simulink model "SISO_Example_Sim"  (R2017b)
settings: Solver=ode3  StartTime=0.0  StopTime=tfin  FixedStep=dT  RelTol=1e-3
values from neighbouring files (symbols this model uses):
  A = [-a_p, b_p, 0, 0 ... (first row only)    [SISO_Example.m]    (also in SimVFA.m = A')
  a20 = 1    [SISO_Example.m]
  a21 = 2    [SISO_Example.m]
  a22 = 1    [SISO_Example.m]
  A_cmd = [0,   1 ... (first row only)    [SISO_Example.m]
  A_h = [0,   1 ... (first row only)    [SISO_Example.m]
  A_m = A - b_3 * k'    [SISO_Example.m]
  A_star = A + b_1*psi_star_1' + b_3*psi_star_3'    [SISO_Example.m]
  adapt = 1    [SISO_Example.m]
  B_cmd = [0; om_cmd^2]    [SISO_Example.m]
  b_h = [0; a20/a22]    [SISO_Example.m]
  b_p = 1.5    [SISO_Example.m]
  b_r = [0; 0; 0; -1]    [SISO_Example.m]
  ba_2 = a22 * A * b_3 + a21 * b_3    [SISO_Example.m]
  ba_3 = a22 * b_3    [SISO_Example.m]
  C_cmd = eye(2)    [SISO_Example.m]
  c_h1 = [0; 1]    [SISO_Example.m]
  c_h2 = [-a20/a22; -a21/a22]    [SISO_Example.m]
  cmd_mag = 1    [SISO_Example.m]
  g = 32.2    [VFA_v1.m]
  k = lqr(A, b_3, Q, r)'    [SISO_Example.m]
  l = eps * ba_1 * b_p * om_n^2    [SISO_Example.m]
  lam_star = lam_star_p * lam_star_a    (= 1)    [SISO_Example.m]
  mu = 2    [SISO_Example.m]
  om_n = 2.6    [SISO_Example.m]
  sine_freq = 1    [SISO_Example.m]
  step_time = 1    [SISO_Example.m]
  steps = length(so.tout)    [SISO_Example.m]    (also in SimVFA.m = length(SOO.t_sim))
settings Model: Creator=ben  LastModifiedBy=ben
settings DataIOCC: SaveOutput=off  SignalLogging=off  DSMLogging=off  ReturnWorkspaceOutputs=on  ReturnWorkspaceOutputsName=simout

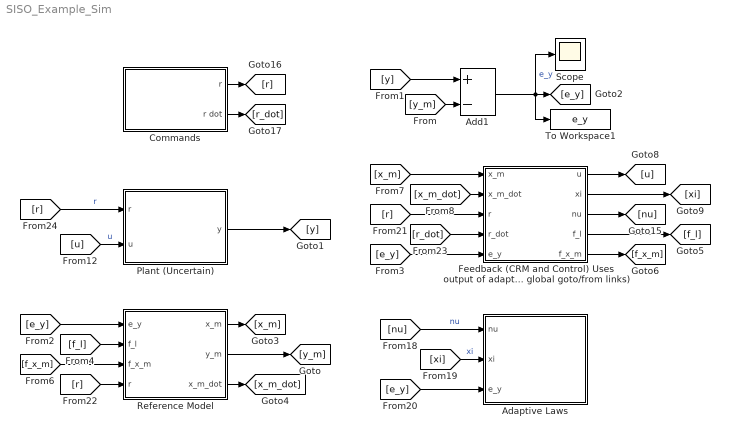
== system SISO_Example_Sim ==
  Adaptive Laws : Subsystem
  Add1 : Sum  Inputs=+-
  Commands : Subsystem
  Feedback (CRM and Control) Uses output of adaptive laws (here via global goto/from links) : Subsystem
  Plant (Uncertain) : Subsystem
  Reference Model : Subsystem
  Scope : Scope
  To Workspace1 : ToWorkspace  VariableName=e_y  SampleTime=-1
  wires:
  [y] -> Add1/1
  [y_m] -> Add1/2
  Add1/1 -> Scope/1, To Workspace1/1, [e_y]  "e_y"
  [e_y] -> Reference Model/1(e_y)
  Reference Model/1(x_m) -> [x_m]
  Reference Model/2(y_m) -> [y_m]
  Reference Model/3(x_m_dot) -> [x_m_dot]
  [f_l] -> Reference Model/2(f_l)
  [f_x_m] -> Reference Model/3(f_x_m)
  [nu] -> Adaptive Laws/1(nu)  "nu"
  [xi] -> Adaptive Laws/2(xi)  "xi"
  [e_y] -> Adaptive Laws/3(e_y)
  Commands/1(r) -> [r]
  Commands/2(r dot) -> [r_dot]
  [r] -> Reference Model/4(r)
  [r] -> Plant (Uncertain)/1(r)  "r"
  [u] -> Plant (Uncertain)/2(u)  "u"
  Plant (Uncertain)/1(y) -> [y]
  [x_m] -> Feedback (CRM and Control) Uses output of adaptive laws (here via global goto/from links)/1(x_m)
  [x_m_dot] -> Feedback (CRM and Control) Uses output of adaptive laws (here via global goto/from links)/2(x_m_dot)
  [r] -> Feedback (CRM and Control) Uses output of adaptive laws (here via global goto/from links)/3(r)
  [r_dot] -> Feedback (CRM and Control) Uses output of adaptive laws (here via global goto/from links)/4(r_dot)
  [e_y] -> Feedback (CRM and Control) Uses output of adaptive laws (here via global goto/from links)/5(e_y)
  Feedback (CRM and Control) Uses output of adaptive laws (here via global goto/from links)/1(u) -> [u]
  Feedback (CRM and Control) Uses output of adaptive laws (here via global goto/from links)/2(xi) -> [xi]
  Feedback (CRM and Control) Uses output of adaptive laws (here via global goto/from links)/3(nu) -> [nu]
  Feedback (CRM and Control) Uses output of adaptive laws (here via global goto/from links)/4(f_l) -> [f_l]
  Feedback (CRM and Control) Uses output of adaptive laws (here via global goto/from links)/5(f_x_m) -> [f_x_m]

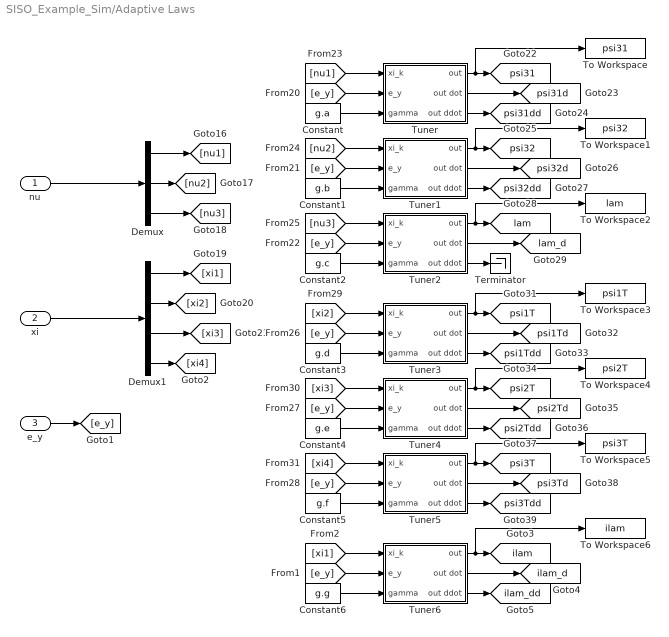
== system SISO_Example_Sim/Adaptive Laws ==
  nu : Inport
  xi : Inport  Port=2
  e_y : Inport  Port=3
  Constant : Constant  Value=g.a
  Constant1 : Constant  Value=g.b
  Constant2 : Constant  Value=g.c
  Constant3 : Constant  Value=g.d
  Constant4 : Constant  Value=g.e
  Constant5 : Constant  Value=g.f
  Constant6 : Constant  Value=g.g
  Demux : Demux  Outputs=[1 1 1]
  Demux1 : Demux  Outputs=[1 4 4 4]
  Terminator : Terminator
  To Workspace : ToWorkspace  VariableName=psi31  SampleTime=-1
  To Workspace1 : ToWorkspace  VariableName=psi32  SampleTime=-1
  To Workspace2 : ToWorkspace  VariableName=lam  SampleTime=-1
  To Workspace3 : ToWorkspace  VariableName=psi1T  SampleTime=-1
  To Workspace4 : ToWorkspace  VariableName=psi2T  SampleTime=-1
  To Workspace5 : ToWorkspace  VariableName=psi3T  SampleTime=-1
  To Workspace6 : ToWorkspace  VariableName=ilam  SampleTime=-1
  Tuner : Subsystem
  Tuner1 : Subsystem
  Tuner2 : Subsystem
  Tuner3 : Subsystem
  Tuner4 : Subsystem
  Tuner5 : Subsystem
  Tuner6 : Subsystem
  tag scope: ilam=global, ilam_d=global, ilam_dd=global, lam=global, lam_d=global, psi1T=global, psi1Td=global, psi1Tdd=global, psi2T=global, psi2Td=global, psi2Tdd=global, psi31=global, psi31d=global, psi31dd=global, psi32=global, psi32d=global, psi32dd=global, psi3T=global, psi3Td=global, psi3Tdd=global
  wires:
  Tuner3/3(out ddot) -> [psi1Tdd]
  nu/1 -> Demux/1
  Tuner5/2(out dot) -> [psi3Td]
  Demux/1 -> [nu1]
  Tuner4/1(out) -> To Workspace4/1, [psi2T]
  [nu1] -> Tuner/1(xi_k)
  [nu2] -> Tuner1/1(xi_k)
  [e_y] -> Tuner1/2(e_y)
  [e_y] -> Tuner/2(e_y)
  Tuner2/1(out) -> To Workspace2/1, [lam]
  Tuner/3(out ddot) -> [psi31dd]
  Tuner1/3(out ddot) -> [psi32dd]
  Tuner3/1(out) -> To Workspace3/1, [psi1T]
  Demux/3 -> [nu3]
  [xi4] -> Tuner5/1(xi_k)
  [e_y] -> Tuner3/2(e_y)
  Tuner/2(out dot) -> [psi31d]
  Tuner1/2(out dot) -> [psi32d]
  [xi2] -> Tuner3/1(xi_k)
  [e_y] -> Tuner5/2(e_y)
  [e_y] -> Tuner4/2(e_y)
  [xi3] -> Tuner4/1(xi_k)
  xi/1 -> Demux1/1
  [e_y] -> Tuner2/2(e_y)
  Tuner2/3(out ddot) -> Terminator/1
  Demux1/3 -> [xi3]
  Tuner5/3(out ddot) -> [psi3Tdd]
  [nu3] -> Tuner2/1(xi_k)
  Tuner/1(out) -> To Workspace/1, [psi31]
  Tuner2/2(out dot) -> [lam_d]
  Tuner4/2(out dot) -> [psi2Td]
  Tuner1/1(out) -> To Workspace1/1, [psi32]
  Tuner4/3(out ddot) -> [psi2Tdd]
  Demux1/1 -> [xi1]
  Demux1/2 -> [xi2]
  Demux/2 -> [nu2]
  Tuner3/2(out dot) -> [psi1Td]
  e_y/1 -> [e_y]
  Tuner5/1(out) -> To Workspace5/1, [psi3T]
  Demux1/4 -> [xi4]
  [xi1] -> Tuner6/1(xi_k)
  [e_y] -> Tuner6/2(e_y)
  Tuner6/1(out) -> To Workspace6/1, [ilam]
  Tuner6/3(out ddot) -> [ilam_dd]
  Tuner6/2(out dot) -> [ilam_d]
  Constant/1 -> Tuner/3(gamma)
  Constant1/1 -> Tuner1/3(gamma)
  Constant2/1 -> Tuner2/3(gamma)
  Constant3/1 -> Tuner3/3(gamma)
  Constant4/1 -> Tuner4/3(gamma)
  Constant5/1 -> Tuner5/3(gamma)
  Constant6/1 -> Tuner6/3(gamma)

== system SISO_Example_Sim/Commands ==
  Command Filter : StateSpace  A=A_cmd  B=B_cmd  C=C_cmd  D=[0; 0]  InitialCondition=0
  Constant : Constant  Value=steps
  Constant1 : Constant  Value=cmd_mag/2
  Demux : Demux  Outputs=[1 1]
  Pulse Generator : DiscretePulseGenerator  PulseType=Time based  Amplitude=cmd_mag  Period=2*step_time  PulseWidth=50
  Sine Wave : Sin  Amplitude=cmd_mag  Frequency=sine_freq  SampleTime=0
  Sum : Sum  Inputs=-+|
  Switch : Switch  Criteria=u2 ~= 0
  To Workspace1 : ToWorkspace  VariableName=r_dot  SampleTime=-1
  To Workspace3 : ToWorkspace  VariableName=r  SampleTime=-1
  r : Outport
  r dot : Outport  Port=2
  wires:
  Demux/2 -> To Workspace1/1, r dot/1  "r dot"
  Command Filter/1 -> Demux/1
  Demux/1 -> To Workspace3/1, r/1  "r (alternatively z_cmd)"
  Constant/1 -> Switch/2
  Switch/1 -> Command Filter/1
  Sum/1 -> Switch/1
  Sine Wave/1 -> Switch/3
  Pulse Generator/1 -> Sum/2
  Constant1/1 -> Sum/1

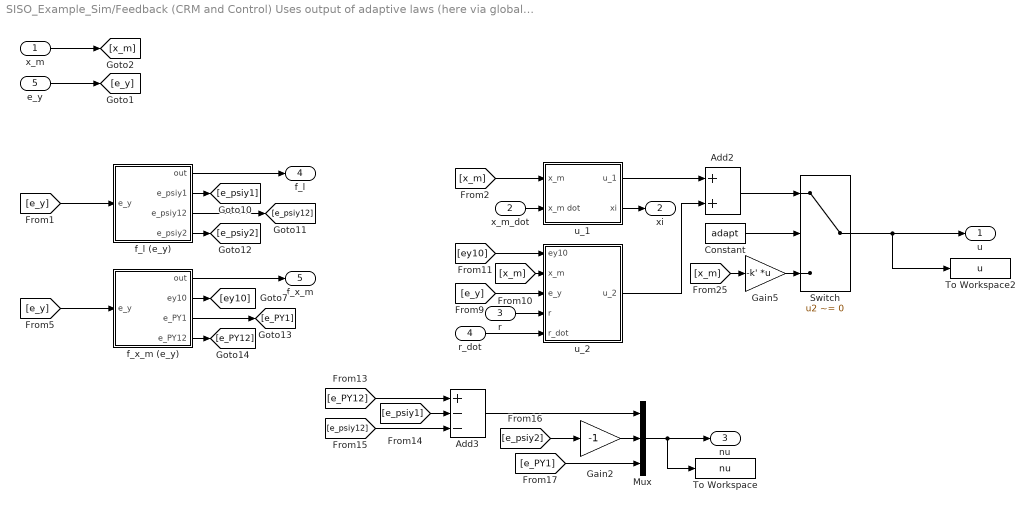
== system SISO_Example_Sim/Feedback (CRM and Control) Uses output of adaptive laws (here via global goto//from links) ==
  x_m : Inport
  x_m_dot : Inport  Port=2
  r : Inport  Port=3
  r_dot : Inport  Port=4
  e_y : Inport  Port=5
  Add2 : Sum
  Add3 : Sum  Inputs=+--
  Constant : Constant  Value=adapt
  Gain2 : Gain  Gain=-1
  Gain5 : Gain  Gain=-k'  Multiplication=Matrix(K*u)
  Mux : Mux  Inputs=[1 1 1]
  Switch : Switch  Criteria=u2 ~= 0
  To Workspace : ToWorkspace  VariableName=nu  SampleTime=-1
  To Workspace2 : ToWorkspace  VariableName=u  SampleTime=-1
  f_l (e_y) : Subsystem
  f_x_m (e_y) : Subsystem
  u_1 : Subsystem
  u_2 : Subsystem
  u : Outport
  xi : Outport  Port=2
  nu : Outport  Port=3
  f_l : Outport  Port=4
  f_x_m : Outport  Port=5
  wires:
  [e_PY1] -> Mux/3
  Gain2/1 -> Mux/2
  [e_psiy2] -> Gain2/1
  [e_psiy12] -> Add3/3
  [e_psiy1] -> Add3/2
  [e_PY12] -> Add3/1
  Add3/1 -> Mux/1
  f_x_m (e_y)/4(e_PY12) -> [e_PY12]
  f_x_m (e_y)/3(e_PY1) -> [e_PY1]
  f_l (e_y)/4(e_psiy2) -> [e_psiy2]
  f_l (e_y)/3(e_psiy12) -> [e_psiy12]
  f_l (e_y)/2(e_psiy1) -> [e_psiy1]
  u_1/2(xi) -> xi/1
  Switch/1 -> u/1, To Workspace2/1
  u_2/1(u_2) -> Add2/2
  u_1/1(u_1) -> Add2/1
  [ey10] -> u_2/1(ey10)
  [e_y] -> u_2/3(e_y)
  f_x_m (e_y)/2(ey10) -> [ey10]
  x_m_dot/1 -> u_1/2(x_m dot)
  f_x_m (e_y)/1(out) -> f_x_m/1
  [e_y] -> f_x_m (e_y)/1(e_y)
  [x_m] -> u_2/2(x_m)
  f_l (e_y)/1(out) -> f_l/1
  Mux/1 -> nu/1, To Workspace/1
  r/1 -> u_2/4(r)
  r_dot/1 -> u_2/5(r_dot)
  Constant/1 -> Switch/2
  Add2/1 -> Switch/1
  Gain5/1 -> Switch/3
  [x_m] -> Gain5/1
  e_y/1 -> [e_y]
  [e_y] -> f_l (e_y)/1(e_y)
  x_m/1 -> [x_m]
  [x_m] -> u_1/1(x_m)

== system SISO_Example_Sim/Plant (Uncertain) ==
  r : Inport
  u : Inport  Port=2
  Add : Sum  Inputs=+++
  Gain1 : Gain  Gain=lam_star
  Gain3 : Gain  Gain=b_r  Multiplication=Matrix(K*u)
  Gain4 : Gain  Gain=A_star  Multiplication=Matrix(K*u)
  Gain5 : Gain  Gain=c'  Multiplication=Matrix(K*u)
  Integrator : Integrator
  Signal Specification2 : SignalSpecification  Dimensions=[4 1]
  To Workspace3 : ToWorkspace  VariableName=y  SampleTime=-1
  y : Outport
  wires:
  u/1 -> Gain1/1
  Gain5/1 -> y/1, To Workspace3/1
  Add/1 -> Signal Specification2/1  "x_dot"
  Gain4/1 -> Add/1  "(A*) * x"
  Integrator/1 -> Gain4/1, Gain5/1  "x"
  Gain3/1 -> Add/2  "b_r * r"
  r/1 -> Gain3/1
  Signal Specification2/1 -> Integrator/1  "x_dot"
  Gain1/1 -> Add/3

== system SISO_Example_Sim/Reference Model ==
  e_y : Inport
  f_l : Inport  Port=2
  f_x_m : Inport  Port=3
  r : Inport  Port=4
  Add : Sum  Inputs=+++++
  Gain : Gain  Gain=c'  Multiplication=Matrix(K*u)
  Gain1 : Gain  Gain=l  Multiplication=Matrix(K*u)
  Gain2 : Gain  Gain=A_m  Multiplication=Matrix(K*u)
  Gain3 : Gain  Gain=b_r  Multiplication=Matrix(K*u)
  Integrator : Integrator
  Signal Specification2 : SignalSpecification  Dimensions=[4 1]
  To Workspace : ToWorkspace  VariableName=x_m  SampleTime=-1
  To Workspace1 : ToWorkspace  VariableName=y_m  SampleTime=-1
  x_m : Outport
  y_m : Outport  Port=2
  x_m_dot : Outport  Port=3
  wires:
  Gain2/1 -> Add/1  "A_m * x_m"
  f_x_m/1 -> Add/4
  e_y/1 -> Gain1/1
  Gain/1 -> To Workspace1/1, y_m/1  "y_m"
  Gain1/1 -> Add/2  "l * e_y"
  Integrator/1 -> To Workspace/1, x_m/1, Gain2/1, Gain/1  "x_m"
  Signal Specification2/1 -> x_m_dot/1, Integrator/1  "x_m_dot"
  f_l/1 -> Add/3
  Add/1 -> Signal Specification2/1  "x_m_dot"
  Gain3/1 -> Add/5
  r/1 -> Gain3/1

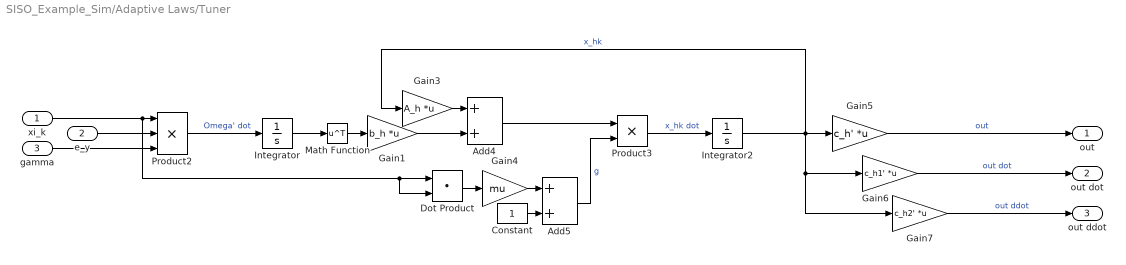
== system SISO_Example_Sim/Adaptive Laws/Tuner ==
  xi_k : Inport
  e_y : Inport  Port=2
  gamma : Inport  Port=3
  Add4 : Sum
  Add5 : Sum
  Constant : Constant
  Dot Product : DotProduct  InputSameDT=on  OutDataTypeStr=Inherit: Inherit via internal rule
  Gain1 : Gain  Gain=b_h  Multiplication=Matrix(K*u)
  Gain3 : Gain  Gain=A_h  Multiplication=Matrix(K*u)
  Gain4 : Gain  Gain=mu
  Gain5 : Gain  Gain=c_h'  Multiplication=Matrix(K*u)
  Gain6 : Gain  Gain=c_h1'  Multiplication=Matrix(K*u)
  Gain7 : Gain  Gain=c_h2'  Multiplication=Matrix(K*u)
  Integrator : Integrator
  Integrator2 : Integrator
  Math Function : Math  Operator=transpose  SaturateOnIntegerOverflow=on
  Product2 : Product  Inputs=3
  Product3 : Product
  out : Outport
  out dot : Outport  Port=2
  out ddot : Outport  Port=3
  wires:
  Constant/1 -> Add5/2
  Math Function/1 -> Gain1/1
  Add4/1 -> Product3/1
  e_y/1 -> Product2/2
  Gain5/1 -> out/1  "out"
  Gain1/1 -> Add4/2
  Product3/1 -> Integrator2/1  "x_hk dot"
  Integrator/1 -> Math Function/1
  Integrator2/1 -> Gain7/1, Gain6/1, Gain5/1, Gain3/1  "x_hk"
  Gain7/1 -> out ddot/1  "out ddot"
  Product2/1 -> Integrator/1  "Omega' dot"
  Add5/1 -> Product3/2  "g"
  xi_k/1 -> Dot Product/2, Dot Product/1, Product2/1
  Gain4/1 -> Add5/1
  Dot Product/1 -> Gain4/1
  Gain3/1 -> Add4/1
  Gain6/1 -> out dot/1  "out dot"
  gamma/1 -> Product2/3

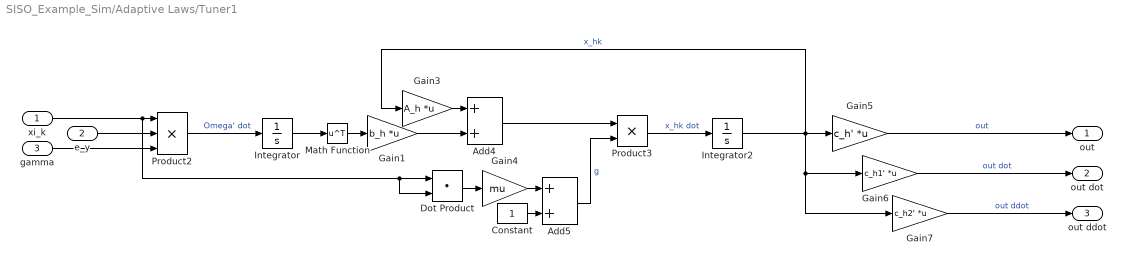
== system SISO_Example_Sim/Adaptive Laws/Tuner1 ==
  xi_k : Inport
  e_y : Inport  Port=2
  gamma : Inport  Port=3
  Add4 : Sum
  Add5 : Sum
  Constant : Constant
  Dot Product : DotProduct  InputSameDT=on  OutDataTypeStr=Inherit: Inherit via internal rule
  Gain1 : Gain  Gain=b_h  Multiplication=Matrix(K*u)
  Gain3 : Gain  Gain=A_h  Multiplication=Matrix(K*u)
  Gain4 : Gain  Gain=mu
  Gain5 : Gain  Gain=c_h'  Multiplication=Matrix(K*u)
  Gain6 : Gain  Gain=c_h1'  Multiplication=Matrix(K*u)
  Gain7 : Gain  Gain=c_h2'  Multiplication=Matrix(K*u)
  Integrator : Integrator
  Integrator2 : Integrator
  Math Function : Math  Operator=transpose  SaturateOnIntegerOverflow=on
  Product2 : Product  Inputs=3
  Product3 : Product
  out : Outport
  out dot : Outport  Port=2
  out ddot : Outport  Port=3
  wires:
  gamma/1 -> Product2/3
  Gain6/1 -> out dot/1  "out dot"
  Gain3/1 -> Add4/1
  Dot Product/1 -> Gain4/1
  Gain4/1 -> Add5/1
  xi_k/1 -> Product2/1, Dot Product/1, Dot Product/2
  Add5/1 -> Product3/2  "g"
  Product2/1 -> Integrator/1  "Omega' dot"
  Gain7/1 -> out ddot/1  "out ddot"
  Integrator2/1 -> Gain3/1, Gain5/1, Gain6/1, Gain7/1  "x_hk"
  Integrator/1 -> Math Function/1
  Product3/1 -> Integrator2/1  "x_hk dot"
  Gain1/1 -> Add4/2
  Gain5/1 -> out/1  "out"
  e_y/1 -> Product2/2
  Add4/1 -> Product3/1
  Math Function/1 -> Gain1/1
  Constant/1 -> Add5/2

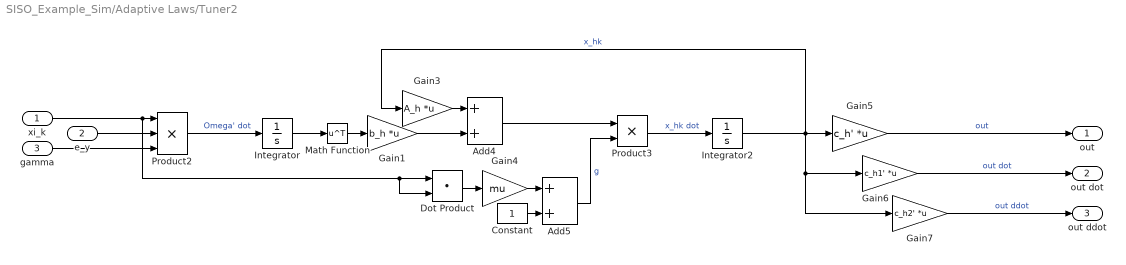
== system SISO_Example_Sim/Adaptive Laws/Tuner2 ==
  xi_k : Inport
  e_y : Inport  Port=2
  gamma : Inport  Port=3
  Add4 : Sum
  Add5 : Sum
  Constant : Constant
  Dot Product : DotProduct  InputSameDT=on  OutDataTypeStr=Inherit: Inherit via internal rule
  Gain1 : Gain  Gain=b_h  Multiplication=Matrix(K*u)
  Gain3 : Gain  Gain=A_h  Multiplication=Matrix(K*u)
  Gain4 : Gain  Gain=mu
  Gain5 : Gain  Gain=c_h'  Multiplication=Matrix(K*u)
  Gain6 : Gain  Gain=c_h1'  Multiplication=Matrix(K*u)
  Gain7 : Gain  Gain=c_h2'  Multiplication=Matrix(K*u)
  Integrator : Integrator
  Integrator2 : Integrator  InitialCondition=[1; 0]
  Math Function : Math  Operator=transpose  SaturateOnIntegerOverflow=on
  Product2 : Product  Inputs=3
  Product3 : Product
  out : Outport
  out dot : Outport  Port=2
  out ddot : Outport  Port=3
  wires:
  Constant/1 -> Add5/2
  Math Function/1 -> Gain1/1
  Add4/1 -> Product3/1
  e_y/1 -> Product2/2
  Gain5/1 -> out/1  "out"
  Gain1/1 -> Add4/2
  Product3/1 -> Integrator2/1  "x_hk dot"
  Integrator/1 -> Math Function/1
  Integrator2/1 -> Gain7/1, Gain6/1, Gain5/1, Gain3/1  "x_hk"
  Gain7/1 -> out ddot/1  "out ddot"
  Product2/1 -> Integrator/1  "Omega' dot"
  Add5/1 -> Product3/2  "g"
  xi_k/1 -> Dot Product/2, Dot Product/1, Product2/1
  Gain4/1 -> Add5/1
  Dot Product/1 -> Gain4/1
  Gain3/1 -> Add4/1
  Gain6/1 -> out dot/1  "out dot"
  gamma/1 -> Product2/3

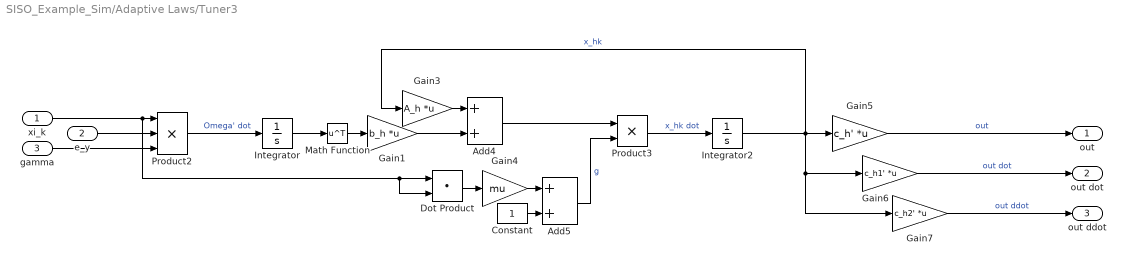
== system SISO_Example_Sim/Adaptive Laws/Tuner3 ==
  xi_k : Inport
  e_y : Inport  Port=2
  gamma : Inport  Port=3
  Add4 : Sum
  Add5 : Sum
  Constant : Constant
  Dot Product : DotProduct  InputSameDT=on  OutDataTypeStr=Inherit: Inherit via internal rule
  Gain1 : Gain  Gain=b_h  Multiplication=Matrix(K*u)
  Gain3 : Gain  Gain=A_h  Multiplication=Matrix(K*u)
  Gain4 : Gain  Gain=mu
  Gain5 : Gain  Gain=c_h'  Multiplication=Matrix(K*u)
  Gain6 : Gain  Gain=c_h1'  Multiplication=Matrix(K*u)
  Gain7 : Gain  Gain=c_h2'  Multiplication=Matrix(K*u)
  Integrator : Integrator
  Integrator2 : Integrator
  Math Function : Math  Operator=transpose  SaturateOnIntegerOverflow=on
  Product2 : Product  Inputs=3
  Product3 : Product
  out : Outport
  out dot : Outport  Port=2
  out ddot : Outport  Port=3
  wires:
  gamma/1 -> Product2/3
  Gain6/1 -> out dot/1  "out dot"
  Gain3/1 -> Add4/1
  Dot Product/1 -> Gain4/1
  Gain4/1 -> Add5/1
  xi_k/1 -> Product2/1, Dot Product/1, Dot Product/2
  Add5/1 -> Product3/2  "g"
  Product2/1 -> Integrator/1  "Omega' dot"
  Gain7/1 -> out ddot/1  "out ddot"
  Integrator2/1 -> Gain3/1, Gain5/1, Gain6/1, Gain7/1  "x_hk"
  Integrator/1 -> Math Function/1
  Product3/1 -> Integrator2/1  "x_hk dot"
  Gain1/1 -> Add4/2
  Gain5/1 -> out/1  "out"
  e_y/1 -> Product2/2
  Add4/1 -> Product3/1
  Math Function/1 -> Gain1/1
  Constant/1 -> Add5/2

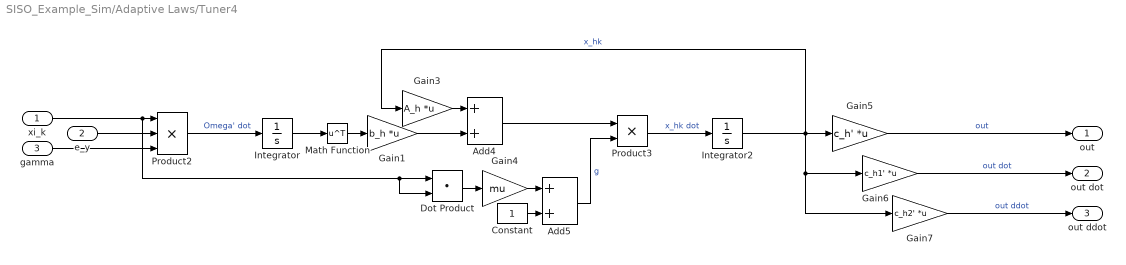
== system SISO_Example_Sim/Adaptive Laws/Tuner4 ==
  xi_k : Inport
  e_y : Inport  Port=2
  gamma : Inport  Port=3
  Add4 : Sum
  Add5 : Sum
  Constant : Constant
  Dot Product : DotProduct  InputSameDT=on  OutDataTypeStr=Inherit: Inherit via internal rule
  Gain1 : Gain  Gain=b_h  Multiplication=Matrix(K*u)
  Gain3 : Gain  Gain=A_h  Multiplication=Matrix(K*u)
  Gain4 : Gain  Gain=mu
  Gain5 : Gain  Gain=c_h'  Multiplication=Matrix(K*u)
  Gain6 : Gain  Gain=c_h1'  Multiplication=Matrix(K*u)
  Gain7 : Gain  Gain=c_h2'  Multiplication=Matrix(K*u)
  Integrator : Integrator
  Integrator2 : Integrator
  Math Function : Math  Operator=transpose  SaturateOnIntegerOverflow=on
  Product2 : Product  Inputs=3
  Product3 : Product
  out : Outport
  out dot : Outport  Port=2
  out ddot : Outport  Port=3
  wires:
  Constant/1 -> Add5/2
  Math Function/1 -> Gain1/1
  Add4/1 -> Product3/1
  e_y/1 -> Product2/2
  Gain5/1 -> out/1  "out"
  Gain1/1 -> Add4/2
  Product3/1 -> Integrator2/1  "x_hk dot"
  Integrator/1 -> Math Function/1
  Integrator2/1 -> Gain7/1, Gain6/1, Gain5/1, Gain3/1  "x_hk"
  Gain7/1 -> out ddot/1  "out ddot"
  Product2/1 -> Integrator/1  "Omega' dot"
  Add5/1 -> Product3/2  "g"
  xi_k/1 -> Dot Product/2, Dot Product/1, Product2/1
  Gain4/1 -> Add5/1
  Dot Product/1 -> Gain4/1
  Gain3/1 -> Add4/1
  Gain6/1 -> out dot/1  "out dot"
  gamma/1 -> Product2/3

== system SISO_Example_Sim/Adaptive Laws/Tuner5 ==
  xi_k : Inport
  e_y : Inport  Port=2
  gamma : Inport  Port=3
  Add4 : Sum
  Add5 : Sum
  Constant : Constant
  Dot Product : DotProduct  InputSameDT=on  OutDataTypeStr=Inherit: Inherit via internal rule
  Gain1 : Gain  Gain=b_h  Multiplication=Matrix(K*u)
  Gain3 : Gain  Gain=A_h  Multiplication=Matrix(K*u)
  Gain4 : Gain  Gain=mu
  Gain5 : Gain  Gain=c_h'  Multiplication=Matrix(K*u)
  Gain6 : Gain  Gain=c_h1'  Multiplication=Matrix(K*u)
  Gain7 : Gain  Gain=c_h2'  Multiplication=Matrix(K*u)
  Integrator : Integrator
  Integrator2 : Integrator
  Math Function : Math  Operator=transpose  SaturateOnIntegerOverflow=on
  Product2 : Product  Inputs=3
  Product3 : Product
  out : Outport
  out dot : Outport  Port=2
  out ddot : Outport  Port=3
  wires:
  gamma/1 -> Product2/3
  Gain6/1 -> out dot/1  "out dot"
  Gain3/1 -> Add4/1
  Dot Product/1 -> Gain4/1
  Gain4/1 -> Add5/1
  xi_k/1 -> Product2/1, Dot Product/1, Dot Product/2
  Add5/1 -> Product3/2  "g"
  Product2/1 -> Integrator/1  "Omega' dot"
  Gain7/1 -> out ddot/1  "out ddot"
  Integrator2/1 -> Gain3/1, Gain5/1, Gain6/1, Gain7/1  "x_hk"
  Integrator/1 -> Math Function/1
  Product3/1 -> Integrator2/1  "x_hk dot"
  Gain1/1 -> Add4/2
  Gain5/1 -> out/1  "out"
  e_y/1 -> Product2/2
  Add4/1 -> Product3/1
  Math Function/1 -> Gain1/1
  Constant/1 -> Add5/2

== system SISO_Example_Sim/Adaptive Laws/Tuner6 ==
  xi_k : Inport
  e_y : Inport  Port=2
  gamma : Inport  Port=3
  Add4 : Sum
  Add5 : Sum
  Constant : Constant
  Dot Product : DotProduct  InputSameDT=on  OutDataTypeStr=Inherit: Inherit via internal rule
  Gain1 : Gain  Gain=b_h  Multiplication=Matrix(K*u)
  Gain3 : Gain  Gain=A_h  Multiplication=Matrix(K*u)
  Gain4 : Gain  Gain=mu
  Gain5 : Gain  Gain=c_h'  Multiplication=Matrix(K*u)
  Gain6 : Gain  Gain=c_h1'  Multiplication=Matrix(K*u)
  Gain7 : Gain  Gain=c_h2'  Multiplication=Matrix(K*u)
  Integrator : Integrator
  Integrator2 : Integrator  InitialCondition=[1; 0]
  Math Function : Math  Operator=transpose  SaturateOnIntegerOverflow=on
  Product2 : Product  Inputs=3
  Product3 : Product
  out : Outport
  out dot : Outport  Port=2
  out ddot : Outport  Port=3
  wires:
  Constant/1 -> Add5/2
  Math Function/1 -> Gain1/1
  Add4/1 -> Product3/1
  e_y/1 -> Product2/2
  Gain5/1 -> out/1  "out"
  Gain1/1 -> Add4/2
  Product3/1 -> Integrator2/1  "x_hk dot"
  Integrator/1 -> Math Function/1
  Integrator2/1 -> Gain7/1, Gain6/1, Gain5/1, Gain3/1  "x_hk"
  Gain7/1 -> out ddot/1  "out ddot"
  Product2/1 -> Integrator/1  "Omega' dot"
  Add5/1 -> Product3/2  "g"
  xi_k/1 -> Dot Product/2, Dot Product/1, Product2/1
  Gain4/1 -> Add5/1
  Dot Product/1 -> Gain4/1
  Gain3/1 -> Add4/1
  Gain6/1 -> out dot/1  "out dot"
  gamma/1 -> Product2/3

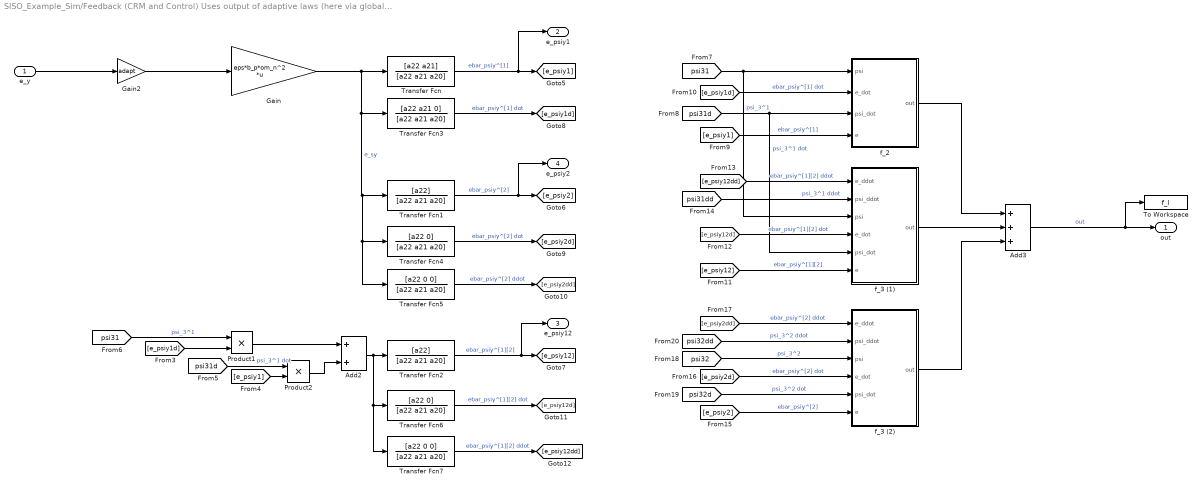
== system SISO_Example_Sim/Feedback (CRM and Control) Uses output of adaptive laws (here via global goto//from links)/f_l (e_y) ==
  e_y : Inport
  Add2 : Sum
  Add3 : Sum  Inputs=+++
  Gain : Gain  Gain=eps*b_p*om_n^2  Multiplication=Matrix(K*u)
  Gain2 : Gain  Gain=adapt
  Product1 : Product
  Product2 : Product
  To Workspace : ToWorkspace  VariableName=f_l  SampleTime=-1
  Transfer Fcn : TransferFcn  Numerator=[a22 a21]  Denominator=[a22 a21 a20]
  Transfer Fcn1 : TransferFcn  Numerator=[a22]  Denominator=[a22 a21 a20]
  Transfer Fcn2 : TransferFcn  Numerator=[a22]  Denominator=[a22 a21 a20]
  Transfer Fcn3 : TransferFcn  Numerator=[a22 a21 0]  Denominator=[a22 a21 a20]
  Transfer Fcn4 : TransferFcn  Numerator=[a22 0]  Denominator=[a22 a21 a20]
  Transfer Fcn5 : TransferFcn  Numerator=[a22 0 0]  Denominator=[a22 a21 a20]
  Transfer Fcn6 : TransferFcn  Numerator=[a22 0]  Denominator=[a22 a21 a20]
  Transfer Fcn7 : TransferFcn  Numerator=[a22 0 0]  Denominator=[a22 a21 a20]
  f_2 : Subsystem
  f_3 (1) : Subsystem
  f_3 (2) : Subsystem
  out : Outport
  e_psiy1 : Outport  Port=2
  e_psiy12 : Outport  Port=3
  e_psiy2 : Outport  Port=4
  wires:
  [e_psiy12dd] -> f_3 (1)/1(e_ddot)  "ebar_psiy^[1][2] ddot"
  Transfer Fcn7/1 -> [e_psiy12dd]  "ebar_psiy^[1][2] ddot"
  f_3 (1)/1(out) -> Add3/2
  [psi31d] -> f_2/3(psi_dot), f_3 (1)/5(psi_dot)  "psi_3^1 dot"
  [psi31] -> f_2/1(psi), f_3 (1)/3(psi)  "psi_3^1"
  f_2/1(out) -> Add3/1
  [psi31] -> Product1/1  "psi_3^1"
  Transfer Fcn1/1 -> e_psiy2/1, [e_psiy2]  "ebar_psiy^[2]"
  [e_psiy2dd] -> f_3 (2)/1(e_ddot)  "ebar_psiy^[2] ddot"
  [psi32dd] -> f_3 (2)/2(psi_ddot)  "psi_3^2 ddot"
  [psi32d] -> f_3 (2)/5(psi_dot)  "psi_3^2 dot"
  [e_psiy12d] -> f_3 (1)/4(e_dot)  "ebar_psiy^[1][2] dot"
  [e_psiy1d] -> f_2/2(e_dot)  "ebar_psiy^[1] dot"
  f_3 (2)/1(out) -> Add3/3
  Transfer Fcn4/1 -> [e_psiy2d]  "ebar_psiy^[2] dot"
  [psi31d] -> Product2/1  "psi_3^1 dot"
  Add3/1 -> To Workspace/1, out/1  "out"
  Transfer Fcn6/1 -> [e_psiy12d]  "ebar_psiy^[1][2] dot"
  Transfer Fcn2/1 -> e_psiy12/1, [e_psiy12]  "ebar_psiy^[1][2]"
  [e_psiy2] -> f_3 (2)/6(e)  "ebar_psiy^[2]"
  Gain/1 -> Transfer Fcn3/1, Transfer Fcn5/1, Transfer Fcn4/1, Transfer Fcn1/1, Transfer Fcn/1  "e_sy"
  Add2/1 -> Transfer Fcn7/1, Transfer Fcn6/1, Transfer Fcn2/1
  [e_psiy1] -> Product2/2
  [psi31dd] -> f_3 (1)/2(psi_ddot)  "psi_3^1 ddot"
  Product1/1 -> Add2/1
  [e_psiy1d] -> Product1/2
  Product2/1 -> Add2/2
  Transfer Fcn3/1 -> [e_psiy1d]  "ebar_psiy^[1] dot"
  [e_psiy12] -> f_3 (1)/6(e)  "ebar_psiy^[1][2]"
  Transfer Fcn/1 -> e_psiy1/1, [e_psiy1]  "ebar_psiy^[1]"
  [psi32] -> f_3 (2)/3(psi)  "psi_3^2"
  [e_psiy2d] -> f_3 (2)/4(e_dot)  "ebar_psiy^[2] dot"
  e_y/1 -> Gain2/1
  [e_psiy1] -> f_2/4(e)  "ebar_psiy^[1]"
  Transfer Fcn5/1 -> [e_psiy2dd]  "ebar_psiy^[2] ddot"
  Gain2/1 -> Gain/1

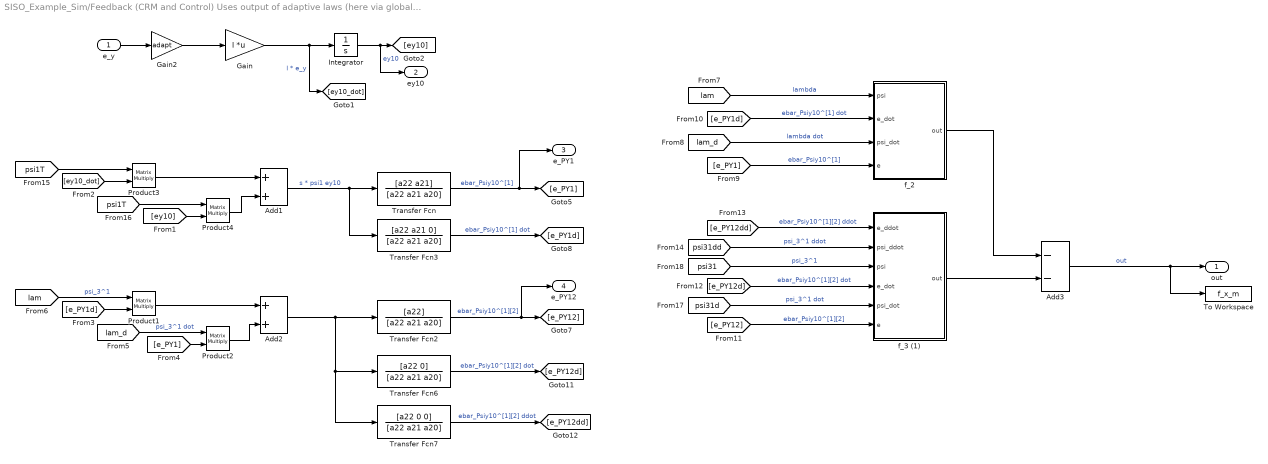
== system SISO_Example_Sim/Feedback (CRM and Control) Uses output of adaptive laws (here via global goto//from links)/f_x_m (e_y) ==
  e_y : Inport
  Add1 : Sum
  Add2 : Sum
  Add3 : Sum  Inputs=--
  Gain : Gain  Gain=l  Multiplication=Matrix(K*u)
  Gain2 : Gain  Gain=adapt
  Integrator : Integrator
  Product{1..4} (4 alike) : Product  Multiplication=Matrix(*)
  To Workspace : ToWorkspace  VariableName=f_x_m  SampleTime=-1
  Transfer Fcn : TransferFcn  Numerator=[a22 a21]  Denominator=[a22 a21 a20]
  Transfer Fcn2 : TransferFcn  Numerator=[a22]  Denominator=[a22 a21 a20]
  Transfer Fcn3 : TransferFcn  Numerator=[a22 a21 0]  Denominator=[a22 a21 a20]
  Transfer Fcn6 : TransferFcn  Numerator=[a22 0]  Denominator=[a22 a21 a20]
  Transfer Fcn7 : TransferFcn  Numerator=[a22 0 0]  Denominator=[a22 a21 a20]
  f_2 : Subsystem
  f_3 (1) : Subsystem
  out : Outport
  ey10 : Outport  Port=2
  e_PY1 : Outport  Port=3
  e_PY12 : Outport  Port=4
  wires:
  [e_PY12dd] -> f_3 (1)/1(e_ddot)  "ebar_Psiy10^[1][2] ddot"
  Transfer Fcn7/1 -> [e_PY12dd]  "ebar_Psiy10^[1][2] ddot"
  f_3 (1)/1(out) -> Add3/2
  [lam_d] -> f_2/3(psi_dot)  "lambda dot"
  [lam] -> f_2/1(psi)  "lambda"
  f_2/1(out) -> Add3/1
  [lam] -> Product1/1  "psi_3^1"
  [e_PY12d] -> f_3 (1)/4(e_dot)  "ebar_Psiy10^[1][2] dot"
  [e_PY1d] -> f_2/2(e_dot)  "ebar_Psiy10^[1] dot"
  [lam_d] -> Product2/1  "psi_3^1 dot"
  Add3/1 -> To Workspace/1, out/1  "out"
  Transfer Fcn6/1 -> [e_PY12d]  "ebar_Psiy10^[1][2] dot"
  Transfer Fcn2/1 -> e_PY12/1, [e_PY12]  "ebar_Psiy10^[1][2]"
  Gain/1 -> [ey10_dot], Integrator/1  "l * e_y"
  Add2/1 -> Transfer Fcn2/1, Transfer Fcn6/1, Transfer Fcn7/1
  [e_PY1] -> Product2/2
  [psi31dd] -> f_3 (1)/2(psi_ddot)  "psi_3^1 ddot"
  Product1/1 -> Add2/1
  [e_PY1d] -> Product1/2
  Product2/1 -> Add2/2
  Transfer Fcn3/1 -> [e_PY1d]  "ebar_Psiy10^[1] dot"
  [e_PY12] -> f_3 (1)/6(e)  "ebar_Psiy10^[1][2]"
  Transfer Fcn/1 -> [e_PY1], e_PY1/1  "ebar_Psiy10^[1]"
  e_y/1 -> Gain2/1
  [e_PY1] -> f_2/4(e)  "ebar_Psiy10^[1]"
  Add1/1 -> Transfer Fcn3/1, Transfer Fcn/1  "s * psi1 ey10"
  Integrator/1 -> ey10/1, [ey10]  "ey10"
  Product4/1 -> Add1/2
  Product3/1 -> Add1/1
  [ey10] -> Product4/2
  [ey10_dot] -> Product3/2
  [psi1T] -> Product3/1
  [psi1T] -> Product4/1
  [psi31d] -> f_3 (1)/5(psi_dot)  "psi_3^1 dot"
  [psi31] -> f_3 (1)/3(psi)  "psi_3^1"
  Gain2/1 -> Gain/1

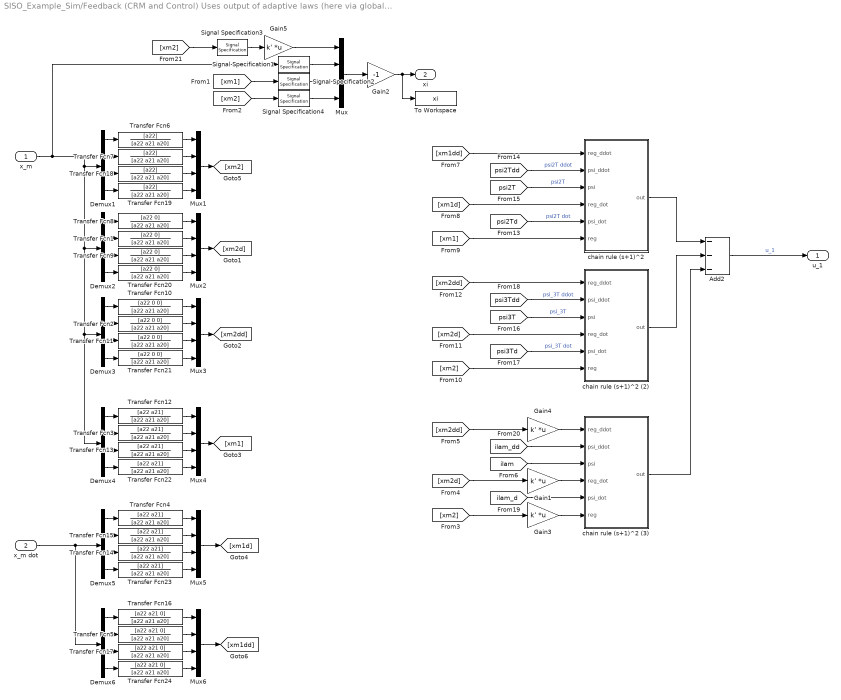
== system SISO_Example_Sim/Feedback (CRM and Control) Uses output of adaptive laws (here via global goto//from links)/u_1 ==
  x_m : Inport
  x_m dot : Inport  Port=2
  Add2 : Sum  Inputs=---
  Demux{1..6} (6 alike) : Demux  Outputs=[1 1 1 1]
  Gain{1,3..5} (4 alike) : Gain  Gain=k'  Multiplication=Matrix(K*u)
  Gain2 : Gain  Gain=-1
  Mux : Mux  Inputs=[1 4 4 4]
  Mux{1..6} (6 alike) : Mux  Inputs=[1 1 1 1]
  Signal Specification{1..4} (4 alike) : SignalSpecification  Dimensions=[4 1]
  To Workspace : ToWorkspace  VariableName=xi  SampleTime=-1
  Transfer Fcn{1,8..9,20} (4 alike) : TransferFcn  Numerator=[a22 0]  Denominator=[a22 a21 a20]
  Transfer Fcn{2,10..11,21} (4 alike) : TransferFcn  Numerator=[a22 0 0]  Denominator=[a22 a21 a20]
  Transfer Fcn{3..4,12..15,22..23} (8 alike) : TransferFcn  Numerator=[a22 a21]  Denominator=[a22 a21 a20]
  Transfer Fcn{5,16..17,24} (4 alike) : TransferFcn  Numerator=[a22 a21 0]  Denominator=[a22 a21 a20]
  Transfer Fcn{6..7,18..19} (4 alike) : TransferFcn  Numerator=[a22]  Denominator=[a22 a21 a20]
  chain rule (s+1)^2 : Subsystem
  chain rule (s+1)^2 (2) : Subsystem
  chain rule (s+1)^2 (3) : Subsystem
  u_1 : Outport
  xi : Outport  Port=2
  wires:
  [xm2d] -> chain rule (s+1)^2 (2)/4(reg_dot)
  chain rule (s+1)^2/1(out) -> Add2/1
  [psi3Td] -> chain rule (s+1)^2 (2)/5(psi_dot)  "psi_3T dot"
  [psi2Td] -> chain rule (s+1)^2/5(psi_dot)  "psi2T dot"
  [psi3Tdd] -> chain rule (s+1)^2 (2)/2(psi_ddot)  "psi_3T ddot"
  [xm2dd] -> chain rule (s+1)^2 (2)/1(reg_ddot)
  Add2/1 -> u_1/1  "u_1"
  [xm2] -> chain rule (s+1)^2 (2)/6(reg)
  [psi3T] -> chain rule (s+1)^2 (2)/3(psi)  "psi_3T"
  [xm1d] -> chain rule (s+1)^2/4(reg_dot)
  [xm1] -> chain rule (s+1)^2/6(reg)
  [psi2T] -> chain rule (s+1)^2/3(psi)  "psi2T"
  chain rule (s+1)^2 (2)/1(out) -> Add2/2
  [psi2Tdd] -> chain rule (s+1)^2/2(psi_ddot)  "psi2T ddot"
  [xm1dd] -> chain rule (s+1)^2/1(reg_ddot)
  x_m/1 -> Signal Specification1/1, Demux1/1, Demux4/1, Demux3/1, Demux2/1
  Mux1/1 -> [xm2]
  Mux2/1 -> [xm2d]
  Mux4/1 -> [xm1]
  Mux5/1 -> [xm1d]
  x_m dot/1 -> Demux6/1, Demux5/1
  [xm1] -> Signal Specification2/1
  [xm2] -> Signal Specification4/1
  Mux/1 -> Gain2/1
  Demux1/2 -> Transfer Fcn7/1
  Transfer Fcn7/1 -> Mux1/2
  Demux1/1 -> Transfer Fcn6/1
  Transfer Fcn6/1 -> Mux1/1
  Demux1/3 -> Transfer Fcn18/1
  Transfer Fcn18/1 -> Mux1/3
  Demux2/2 -> Transfer Fcn1/1
  Transfer Fcn1/1 -> Mux2/2
  Demux2/1 -> Transfer Fcn8/1
  Transfer Fcn8/1 -> Mux2/1
  Demux2/3 -> Transfer Fcn9/1
  Transfer Fcn9/1 -> Mux2/3
  Transfer Fcn2/1 -> Mux3/2
  Mux3/1 -> [xm2dd]
  Demux3/2 -> Transfer Fcn2/1
  Demux3/1 -> Transfer Fcn10/1
  Transfer Fcn10/1 -> Mux3/1
  Demux3/3 -> Transfer Fcn11/1
  Transfer Fcn11/1 -> Mux3/3
  Demux4/2 -> Transfer Fcn3/1
  Transfer Fcn3/1 -> Mux4/2
  Demux4/1 -> Transfer Fcn12/1
  Transfer Fcn12/1 -> Mux4/1
  Demux4/3 -> Transfer Fcn13/1
  Transfer Fcn13/1 -> Mux4/3
  Demux5/2 -> Transfer Fcn15/1
  Transfer Fcn15/1 -> Mux5/2
  Demux5/1 -> Transfer Fcn4/1
  Transfer Fcn4/1 -> Mux5/1
  Demux5/3 -> Transfer Fcn14/1
  Transfer Fcn14/1 -> Mux5/3
  Demux6/2 -> Transfer Fcn5/1
  Transfer Fcn5/1 -> Mux6/2
  Mux6/1 -> [xm1dd]
  Demux6/1 -> Transfer Fcn16/1
  Transfer Fcn16/1 -> Mux6/1
  Demux6/3 -> Transfer Fcn17/1
  Transfer Fcn17/1 -> Mux6/3
  Gain2/1 -> To Workspace/1, xi/1
  [xm2dd] -> Gain4/1
  [xm2d] -> Gain1/1
  [xm2] -> Gain3/1
  [ilam_dd] -> chain rule (s+1)^2 (3)/2(psi_ddot)
  [ilam] -> chain rule (s+1)^2 (3)/3(psi)
  [ilam_d] -> chain rule (s+1)^2 (3)/5(psi_dot)
  Gain4/1 -> chain rule (s+1)^2 (3)/1(reg_ddot)
  Gain1/1 -> chain rule (s+1)^2 (3)/4(reg_dot)
  Gain3/1 -> chain rule (s+1)^2 (3)/6(reg)
  Signal Specification2/1 -> Mux/3
  Signal Specification1/1 -> Mux/2
  Signal Specification4/1 -> Mux/4
  [xm2] -> Signal Specification3/1
  Signal Specification3/1 -> Gain5/1
  Gain5/1 -> Mux/1
  chain rule (s+1)^2 (3)/1(out) -> Add2/3
  Demux1/4 -> Transfer Fcn19/1
  Transfer Fcn19/1 -> Mux1/4
  Demux2/4 -> Transfer Fcn20/1
  Transfer Fcn20/1 -> Mux2/4
  Demux3/4 -> Transfer Fcn21/1
  Transfer Fcn21/1 -> Mux3/4
  Demux4/4 -> Transfer Fcn22/1
  Transfer Fcn22/1 -> Mux4/4
  Demux5/4 -> Transfer Fcn23/1
  Transfer Fcn23/1 -> Mux5/4
  Demux6/4 -> Transfer Fcn24/1
  Transfer Fcn24/1 -> Mux6/4

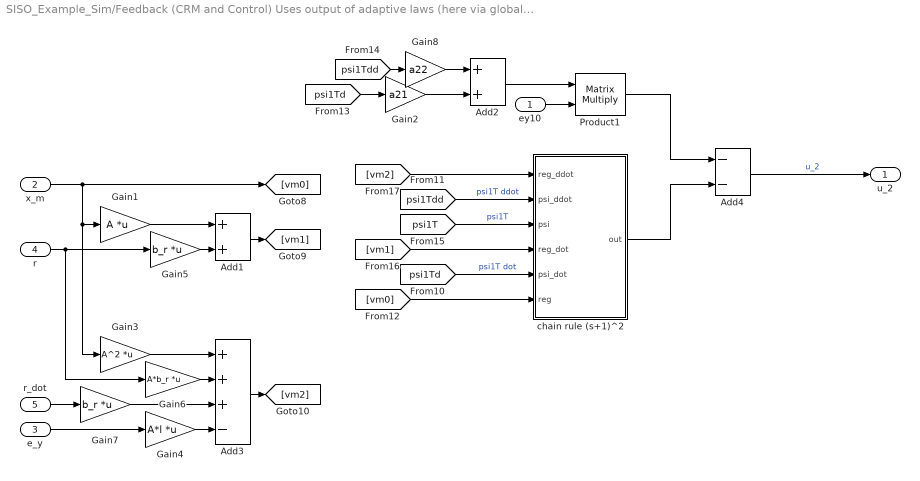
== system SISO_Example_Sim/Feedback (CRM and Control) Uses output of adaptive laws (here via global goto//from links)/u_2 ==
  ey10 : Inport
  x_m : Inport  Port=2
  e_y : Inport  Port=3
  r : Inport  Port=4
  r_dot : Inport  Port=5
  Add1 : Sum
  Add2 : Sum
  Add3 : Sum  Inputs=+++-
  Add4 : Sum  Inputs=--
  Gain1 : Gain  Gain=A  Multiplication=Matrix(K*u)
  Gain2 : Gain  Gain=a21
  Gain3 : Gain  Gain=A^2  Multiplication=Matrix(K*u)
  Gain4 : Gain  Gain=A*l  Multiplication=Matrix(K*u)
  Gain5 : Gain  Gain=b_r  Multiplication=Matrix(K*u)
  Gain6 : Gain  Gain=A*b_r  Multiplication=Matrix(K*u)
  Gain7 : Gain  Gain=b_r  Multiplication=Matrix(K*u)
  Gain8 : Gain  Gain=a22
  Product1 : Product  Multiplication=Matrix(*)
  chain rule (s+1)^2 : Subsystem
  u_2 : Outport
  wires:
  Gain3/1 -> Add3/1
  x_m/1 -> [vm0], Gain3/1, Gain1/1
  Gain2/1 -> Add2/2
  e_y/1 -> Gain4/1
  [vm1] -> chain rule (s+1)^2/4(reg_dot)
  [psi1Td] -> Gain2/1
  Product1/1 -> Add4/1
  Gain1/1 -> Add1/1
  [vm2] -> chain rule (s+1)^2/1(reg_ddot)
  [psi1Td] -> chain rule (s+1)^2/5(psi_dot)  "psi1T dot"
  [psi1T] -> chain rule (s+1)^2/3(psi)  "psi1T"
  Add2/1 -> Product1/1
  [vm0] -> chain rule (s+1)^2/6(reg)
  Add3/1 -> [vm2]
  [psi1Tdd] -> chain rule (s+1)^2/2(psi_ddot)  "psi1T ddot"
  chain rule (s+1)^2/1(out) -> Add4/2
  Gain4/1 -> Add3/4
  Add4/1 -> u_2/1  "u_2"
  ey10/1 -> Product1/2
  Gain8/1 -> Add2/1
  Gain5/1 -> Add1/2
  Add1/1 -> [vm1]
  Gain6/1 -> Add3/2
  Gain7/1 -> Add3/3
  [psi1Tdd] -> Gain8/1
  r/1 -> Gain6/1, Gain5/1
  r_dot/1 -> Gain7/1

== system SISO_Example_Sim/Feedback (CRM and Control) Uses output of adaptive laws (here via global goto//from links)/f_l (e_y)/f_2 ==
  psi : Inport
  e_dot : Inport  Port=2
  psi_dot : Inport  Port=3
  e : Inport  Port=4
  Add2 : Sum
  Add3 : Sum
  Gain : Gain  Gain=ba_2  Multiplication=Matrix(K*u)
  Gain1 : Gain  Gain=ba_3*a20  Multiplication=Matrix(K*u)
  Product1 : Product
  Product2 : Product
  Product3 : Product
  out : Outport
  wires:
  e_dot/1 -> Product1/2
  e/1 -> Product2/2, Product3/2
  Product1/1 -> Add2/1
  Product2/1 -> Add2/2
  psi/1 -> Product3/1, Product1/1
  Gain/1 -> Add3/1
  Gain1/1 -> Add3/2
  psi_dot/1 -> Product2/1
  Add2/1 -> Gain/1
  Add3/1 -> out/1  "out"
  Product3/1 -> Gain1/1

== system SISO_Example_Sim/Feedback (CRM and Control) Uses output of adaptive laws (here via global goto//from links)/f_l (e_y)/f_3 (1) ==
  e_ddot : Inport
  psi_ddot : Inport  Port=2
  psi : Inport  Port=3
  e_dot : Inport  Port=4
  psi_dot : Inport  Port=5
  e : Inport  Port=6
  Add2 : Sum  Inputs=+++
  Add3 : Sum
  Add4 : Sum  Inputs=+++
  Gain1 : Gain  Gain=2
  Gain2 : Gain  Gain=a21
  Gain3 : Gain  Gain=ba_3  Multiplication=Matrix(K*u)
  Gain4 : Gain  Gain=a22
  Gain5 : Gain  Gain=a20
  Product{,1..5} (6 alike) : Product
  out : Outport
  wires:
  Add3/1 -> Gain2/1  "s"
  Product3/1 -> Add3/1
  Product4/1 -> Add3/2
  Gain3/1 -> out/1  "out"
  Product1/1 -> Gain1/1
  e_ddot/1 -> Product/2
  Product5/1 -> Gain5/1  "s^0"
  psi_ddot/1 -> Product2/1
  e_dot/1 -> Product3/2, Product1/2
  Product2/1 -> Add2/3
  e/1 -> Product2/2, Product4/2, Product5/2
  Add2/1 -> Gain4/1  "s^2"
  Gain2/1 -> Add4/2
  Add4/1 -> Gain3/1
  psi_dot/1 -> Product4/1, Product1/1
  psi/1 -> Product3/1, Product5/1, Product/1
  Gain1/1 -> Add2/2
  Product/1 -> Add2/1
  Gain4/1 -> Add4/1
  Gain5/1 -> Add4/3

== system SISO_Example_Sim/Feedback (CRM and Control) Uses output of adaptive laws (here via global goto//from links)/f_l (e_y)/f_3 (2) ==
  e_ddot : Inport
  psi_ddot : Inport  Port=2
  psi : Inport  Port=3
  e_dot : Inport  Port=4
  psi_dot : Inport  Port=5
  e : Inport  Port=6
  Add2 : Sum  Inputs=+++
  Add3 : Sum
  Add4 : Sum  Inputs=+++
  Gain1 : Gain  Gain=2
  Gain2 : Gain  Gain=a21
  Gain3 : Gain  Gain=ba_3  Multiplication=Matrix(K*u)
  Gain4 : Gain  Gain=a22
  Gain5 : Gain  Gain=a20
  Product{,1..5} (6 alike) : Product
  out : Outport
  wires:
  Product/1 -> Add2/1
  Gain1/1 -> Add2/2
  psi/1 -> Product/1, Product5/1, Product3/1
  psi_dot/1 -> Product1/1, Product4/1
  Add4/1 -> Gain3/1
  Gain2/1 -> Add4/2
  Add2/1 -> Gain4/1  "s^2"
  e/1 -> Product5/2, Product4/2, Product2/2
  Product2/1 -> Add2/3
  e_dot/1 -> Product1/2, Product3/2
  psi_ddot/1 -> Product2/1
  Product5/1 -> Gain5/1  "s^0"
  e_ddot/1 -> Product/2
  Product1/1 -> Gain1/1
  Gain3/1 -> out/1  "out"
  Product4/1 -> Add3/2
  Product3/1 -> Add3/1
  Add3/1 -> Gain2/1  "s"
  Gain5/1 -> Add4/3
  Gain4/1 -> Add4/1

== system SISO_Example_Sim/Feedback (CRM and Control) Uses output of adaptive laws (here via global goto//from links)/f_x_m (e_y)/f_2 ==
  psi : Inport
  e_dot : Inport  Port=2
  psi_dot : Inport  Port=3
  e : Inport  Port=4
  Add2 : Sum
  Add3 : Sum
  Gain : Gain  Gain=ba_2  Multiplication=Matrix(K*u)
  Gain1 : Gain  Gain=ba_3*a20  Multiplication=Matrix(K*u)
  Product1 : Product
  Product2 : Product
  Product3 : Product
  out : Outport
  wires:
  e_dot/1 -> Product1/2
  e/1 -> Product2/2, Product3/2
  Product1/1 -> Add2/1
  Product2/1 -> Add2/2
  psi/1 -> Product3/1, Product1/1
  Gain/1 -> Add3/1
  Gain1/1 -> Add3/2
  psi_dot/1 -> Product2/1
  Add2/1 -> Gain/1
  Add3/1 -> out/1  "out"
  Product3/1 -> Gain1/1

== system SISO_Example_Sim/Feedback (CRM and Control) Uses output of adaptive laws (here via global goto//from links)/f_x_m (e_y)/f_3 (1) ==
  e_ddot : Inport
  psi_ddot : Inport  Port=2
  psi : Inport  Port=3
  e_dot : Inport  Port=4
  psi_dot : Inport  Port=5
  e : Inport  Port=6
  Add2 : Sum  Inputs=+++
  Add3 : Sum
  Add4 : Sum  Inputs=+++
  Gain1 : Gain  Gain=2
  Gain2 : Gain  Gain=a21
  Gain3 : Gain  Gain=ba_3  Multiplication=Matrix(K*u)
  Gain4 : Gain  Gain=a22
  Gain5 : Gain  Gain=a20
  Product{,1..5} (6 alike) : Product
  out : Outport
  wires:
  Add3/1 -> Gain2/1  "s"
  Product3/1 -> Add3/1
  Product4/1 -> Add3/2
  Gain3/1 -> out/1  "out"
  Product1/1 -> Gain1/1
  e_ddot/1 -> Product/2
  Product5/1 -> Gain5/1  "s^0"
  psi_ddot/1 -> Product2/1
  e_dot/1 -> Product3/2, Product1/2
  Product2/1 -> Add2/3
  e/1 -> Product2/2, Product4/2, Product5/2
  Add2/1 -> Gain4/1  "s^2"
  Gain2/1 -> Add4/2
  Add4/1 -> Gain3/1
  psi_dot/1 -> Product4/1, Product1/1
  psi/1 -> Product3/1, Product5/1, Product/1
  Gain1/1 -> Add2/2
  Product/1 -> Add2/1
  Gain5/1 -> Add4/3
  Gain4/1 -> Add4/1

== system SISO_Example_Sim/Feedback (CRM and Control) Uses output of adaptive laws (here via global goto//from links)/u_1/chain rule (s+1)^2 ==
  reg_ddot : Inport
  psi_ddot : Inport  Port=2
  psi : Inport  Port=3
  reg_dot : Inport  Port=4
  psi_dot : Inport  Port=5
  reg : Inport  Port=6
  Add2 : Sum  Inputs=+++
  Add3 : Sum
  Add4 : Sum  Inputs=+++
  Gain1 : Gain  Gain=2
  Gain2 : Gain  Gain=a21
  Gain4 : Gain  Gain=a22
  Gain5 : Gain  Gain=a20
  Product{,1..5} (6 alike) : Product  Multiplication=Matrix(*)
  out : Outport
  wires:
  Add3/1 -> Gain2/1  "s"
  Product3/1 -> Add3/1
  Product4/1 -> Add3/2
  Add4/1 -> out/1  "out"
  Product1/1 -> Gain1/1
  reg_ddot/1 -> Product/2
  Product5/1 -> Gain5/1  "s^0"
  psi_ddot/1 -> Product2/1
  reg_dot/1 -> Product3/2, Product1/2
  Product2/1 -> Add2/3
  reg/1 -> Product2/2, Product4/2, Product5/2
  Add2/1 -> Gain4/1  "s^2"
  Gain2/1 -> Add4/2
  psi_dot/1 -> Product4/1, Product1/1
  psi/1 -> Product3/1, Product5/1, Product/1
  Gain1/1 -> Add2/2
  Product/1 -> Add2/1
  Gain4/1 -> Add4/1
  Gain5/1 -> Add4/3

== system SISO_Example_Sim/Feedback (CRM and Control) Uses output of adaptive laws (here via global goto//from links)/u_1/chain rule (s+1)^2 (2) ==
  reg_ddot : Inport
  psi_ddot : Inport  Port=2
  psi : Inport  Port=3
  reg_dot : Inport  Port=4
  psi_dot : Inport  Port=5
  reg : Inport  Port=6
  Add2 : Sum  Inputs=+++
  Add3 : Sum
  Add4 : Sum  Inputs=+++
  Gain1 : Gain  Gain=2
  Gain2 : Gain  Gain=a21
  Gain4 : Gain  Gain=a22
  Gain5 : Gain  Gain=a20
  Product{,1..5} (6 alike) : Product  Multiplication=Matrix(*)
  out : Outport
  wires:
  Add3/1 -> Gain2/1  "s"
  Product3/1 -> Add3/1
  Product4/1 -> Add3/2
  Add4/1 -> out/1  "out"
  Product1/1 -> Gain1/1
  reg_ddot/1 -> Product/2
  Product5/1 -> Gain5/1  "s^0"
  psi_ddot/1 -> Product2/1
  reg_dot/1 -> Product3/2, Product1/2
  Product2/1 -> Add2/3
  reg/1 -> Product2/2, Product4/2, Product5/2
  Add2/1 -> Gain4/1  "s^2"
  Gain2/1 -> Add4/2
  psi_dot/1 -> Product4/1, Product1/1
  psi/1 -> Product3/1, Product5/1, Product/1
  Gain1/1 -> Add2/2
  Product/1 -> Add2/1
  Gain5/1 -> Add4/3
  Gain4/1 -> Add4/1

== system SISO_Example_Sim/Feedback (CRM and Control) Uses output of adaptive laws (here via global goto//from links)/u_1/chain rule (s+1)^2 (3) ==
  reg_ddot : Inport
  psi_ddot : Inport  Port=2
  psi : Inport  Port=3
  reg_dot : Inport  Port=4
  psi_dot : Inport  Port=5
  reg : Inport  Port=6
  Add2 : Sum  Inputs=+++
  Add3 : Sum
  Add4 : Sum  Inputs=+++
  Gain1 : Gain  Gain=2
  Gain2 : Gain  Gain=a21
  Gain4 : Gain  Gain=a22
  Gain5 : Gain  Gain=a20
  Product{,1..5} (6 alike) : Product  Multiplication=Matrix(*)
  out : Outport
  wires:
  Add3/1 -> Gain2/1  "s"
  Product3/1 -> Add3/1
  Product4/1 -> Add3/2
  Add4/1 -> out/1  "out"
  Product1/1 -> Gain1/1
  reg_ddot/1 -> Product/2
  Product5/1 -> Gain5/1  "s^0"
  psi_ddot/1 -> Product2/1
  reg_dot/1 -> Product3/2, Product1/2
  Product2/1 -> Add2/3
  reg/1 -> Product2/2, Product4/2, Product5/2
  Add2/1 -> Gain4/1  "s^2"
  Gain2/1 -> Add4/2
  psi_dot/1 -> Product1/1, Product4/1
  psi/1 -> Product3/1, Product5/1, Product/1
  Gain1/1 -> Add2/2
  Product/1 -> Add2/1
  Gain4/1 -> Add4/1
  Gain5/1 -> Add4/3

== system SISO_Example_Sim/Feedback (CRM and Control) Uses output of adaptive laws (here via global goto//from links)/u_2/chain rule (s+1)^2 ==
  reg_ddot : Inport
  psi_ddot : Inport  Port=2
  psi : Inport  Port=3
  reg_dot : Inport  Port=4
  psi_dot : Inport  Port=5
  reg : Inport  Port=6
  Add2 : Sum  Inputs=+++
  Add3 : Sum
  Add4 : Sum  Inputs=+++
  Gain1 : Gain  Gain=2
  Gain2 : Gain  Gain=a21
  Gain4 : Gain  Gain=a22
  Gain5 : Gain  Gain=a20
  Product{,1..5} (6 alike) : Product  Multiplication=Matrix(*)
  out : Outport
  wires:
  Add3/1 -> Gain2/1  "s"
  Product3/1 -> Add3/1
  Product4/1 -> Add3/2
  Add4/1 -> out/1  "out"
  Product1/1 -> Gain1/1
  reg_ddot/1 -> Product/2
  Product5/1 -> Gain5/1  "s^0"
  psi_ddot/1 -> Product2/1
  reg_dot/1 -> Product3/2, Product1/2
  Product2/1 -> Add2/3
  reg/1 -> Product2/2, Product4/2, Product5/2
  Add2/1 -> Gain4/1  "s^2"
  Gain2/1 -> Add4/2
  psi_dot/1 -> Product4/1, Product1/1
  psi/1 -> Product3/1, Product5/1, Product/1
  Gain1/1 -> Add2/2
  Product/1 -> Add2/1
  Gain5/1 -> Add4/3
  Gain4/1 -> Add4/1
